simulink model "SRV02_model"  (Simulink 8.0)
settings: Solver=ode45  StartTime=0.0  StopTime=10  RelTol=1e-3
values from neighbouring files (symbols this model uses):
  Beq = 0.0015    [Sve_ikad.m]    (also in matlab.mat)
  Eff_G = 0.9    [Sve_ikad.m]    (also in matlab.mat)
  Eff_M = 0.69    [Sve_ikad.m]    (also in matlab.mat)
  Jeq = 9.785e-5    (= 9.785e-05)    [Sve_ikad.m]    (also in matlab.mat)
  Ke = 0.0076776    [Sve_ikad.m]    (also in matlab.mat)
  Kg = 14    [Sve_ikad.m]    (also in matlab.mat)
  Km = 0.007683    [Sve_ikad.m]    (also in matlab.mat)
  Ra = 2.6    [Sve_ikad.m]    (also in matlab.mat)
settings Model: Creator=Labos  LastModifiedBy=Niko
settings DataIOCC: SignalLoggingSaveFormat=ModelDataLogs
settings DebuggingCC: FcnCallInpInsideContextMsg=UseLocalSettings  StrictBusMsg=Warning
settings GRTTargetCC: CombineOutputUpdateFcns=off  GRTInterface=on

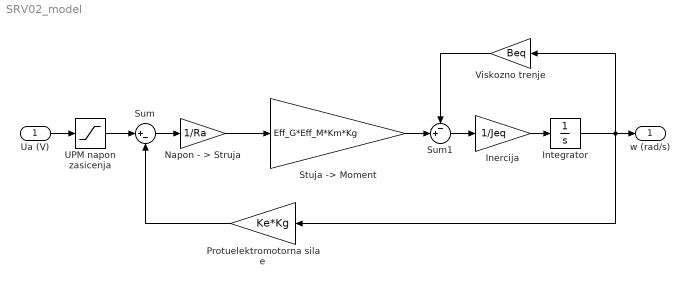
== system SRV02_model ==
  Ua (V) : Inport
  Inercija : Gain  Gain=1/Jeq
  Integrator : Integrator
  Napon - > Struja : Gain  Gain=1/Ra
  Protuelektromotorna sila e : Gain  Gain=Ke*Kg
  "Stuja -> Moment" : Gain  Gain=Eff_G*Eff_M*Km*Kg
  Sum : Sum  Inputs=|+-
  Sum1 : Sum  Inputs=-+|
  UPM napon zasicenja : Saturate  UpperLimit=6  LowerLimit=-6
  Viskozno trenje : Gain  Gain=Beq
  w (rad/s) : Outport
  wires:
  Ua (V)/1 -> UPM napon zasicenja/1
  UPM napon zasicenja/1 -> Sum/1
  Sum/1 -> Napon - > Struja/1
  Sum1/1 -> Inercija/1
  Viskozno trenje/1 -> Sum1/1
  Protuelektromotorna sila e/1 -> Sum/2
  Inercija/1 -> Integrator/1
  Integrator/1 -> Protuelektromotorna sila e/1, Viskozno trenje/1, w (rad/s)/1
  Napon - > Struja/1 -> "Stuja -> Moment"/1
  "Stuja -> Moment"/1 -> Sum1/2
